simulink model "Electrical_System_2018b_obfs"  (R2019b)
settings: Solver=VariableStepAuto  StartTime=0.0  StopTime=5  RelTol=1e-3  AbsTol=1e-3  EnableMultiTasking=on
InitFcn:
  | Steady_State_Initialisation;
StopFcn:
  | %sscexplore(simlog);
  | %Logging
undefined symbols (not defined in the file): abrlhklxvp, aexgmhuedq, afmfmjnutg, afpphrjpnc, ahuxbyvruc, alarvljztt, amxnyqmnuw, aodrlwvqie, aolhmuplyq, aqpmguuqkg, auesgwirzl, aurophlnng, awamelrhru, ayfhvxflxn, azxkacuhqc, babszerikg, bawhdqanwq, bevoqecvei, bltjvqbchx, bmqsuewujl, bsmyqjfgnf, btvjbsmnve, bywgxqeadw, bziaduxaer, bzmcmdqocb, bzsvyvetat, ccsjnrbsih, cdvenygxwh, cedkrnslhx, cjheorclzs, cjrdshrtqx, ckhavyhcza, ckxewznhlz, cmrcgyiplk, conenicnws, cqkejbgjnn, csfnuwymhe, cunupkhwbh, cwzfvzuxxh, dcadmadufn, dcfponivnv, ddtrqjrhjn, dfhoxvkqas, dfrhtcwpne, dfvomcagjv, djijwylxea, dnmeqksrrm, dnzewbdkaa, dsqcykyxav, dtswwlttmm, ecumpidjtv, edegaywrct, ejjjsmnejc, eknqnehjdz, emvdetzouf, esxbqkbahr, etnkkbreiq, eunoiiiirw, ewewcuedir, fatkfxdhtc ... (+386)
libraries: fl_lib x802, ee_lib x362, fl_ps_legacy_lib x160, nesl_utility x85
(part 22 of 26)

== system Electrical_System_2018b_obfs/Redacted_1221/Redacted_7996/Redacted_9242/Redacted_38/Redacted_8107/Redacted_1499 ==
  Redacted_1372 : ee_lib/Semiconductors & Converters/Diode  ModelType=oeqafphldn  Vf=acjyupqtkx V  Ron=elvzancpcm Ohm  Goff=tujcoycxin S  prmExp=bgjswghdna  I12=bkqlogkrkf A  V12=txryfvebun V  IS=otlkguyesn A  ec=opcxekgwui  I1=zxnbsfujxu A  V1=yojkkxomec V  RS=wnxklyqkqh Ohm  Tmeas=naqktatbix degC  N_series=uibfkpxvyo  N_parallel=fsxsmxmqhq  Rz=rxievfeusi Ohm  BV=qlteerppyi V  C_param=lprewekluz  CJ=zephenugoj pF  CJ0=iofcpdtcpe pF  VJ=weostsqpeg V  Mgrad=dsfoutwajc  Vvec=nvjoneietm V  Cvec=yywdcfvqfn pF  FC=zxojfigesc  Q_param=knpwgwovvc  iRM=iptauvkfjs A  iF=evcrxohzeb A  didt=mfkykpnqxj A/us  trr_factor=dkzjtrbhin  trr=egudynmhcl ns  Qrr=skptoxjvyi s*uA  TT=uuwdjlqntv ns  tau=eybdzjqrqe ns  T_param=pdzhxnzkkw  IS_T2=skzmvmtovf A  I1_T2=bcuatdrmea A  V1_T2=ehajjhlbmz V  Tmeas2=tvtzgdgotp degC  EG_param=cqgdiwgdoz  EG=zrtjxhevif eV  XTI_param=fwomuyxozs  XTI=gvlipjngtx  dBVdT=ivbqiupcvu V/K  Tdevice=masylhgtas degC  i_specify=off  i_priority=None  i=lkqqibkans A  i_nominal_specify=off  i_nominal_unit=A  i_nominal_value=rbdmnlhukn  v_specify=off  v_priority=None  v=qqtssrhlfx V  v_nominal_specify=off  v_nominal_unit=V  v_nominal_value=qvmmnhekqw  i_capacitor_specify=off  i_capacitor_priority=None  i_capacitor=uvyrukywri A  i_capacitor_nominal_specify=off  i_capacitor_nominal_unit=A  i_capacitor_nominal_value=aribpcxhol  v_capacitor_specify=off  v_capacitor_priority=None  v_capacitor=qvaywhhawz V  v_capacitor_nominal_specify=off  v_capacitor_nominal_unit=V  v_capacitor_nominal_value=vctwyhqhyz  power_dissipated_specify=off  power_dissipated_priority=None  power_dissipated=ufpbyxefif W  power_dissipated_nominal_specify=off  power_dissipated_nominal_unit=W  power_dissipated_nominal_value=ncmyqqgdsj  thermal_network_parameterization=czsqgtsyze  Rth=deuanxgwux K/W  Rth_Foster=uzfbyrcyqk K/W  thermal_mass_parameterization=cxaszulvyr  thermal_mass=vusczqtjvo J/K  thermal_mass_Foster=bhxnhdayyv J/K  thermal_time_constant=qwdbemvqjo s  thermal_time_constant_Foster=awjktewxjv s  thermal_mass_initial_temperatures=twqhspyowt degC
      settings: SourceProductName=Simscape Electrical  InternalSimscapePortConfiguration="{\"Bottom\":[],\"Left\":[{\"id\":\"p\",\"label\":\"\",\"type\":\"foundation.electrical.electrical\"},{\"id\":\"H\",\"label\":\"H\",\"type\":\"foundation.thermal.thermal\"}],\"Right\":[{\"id\":\"n\",\"label\":\"\",\"type\":\"foundation.electrical.electrical\"}],\"Top\":[]}"
  Redacted_1419 : ee_lib/Passive/Thermal/Thermal Resistor  R=hrqrqmvbpy K/W  T_specify=off  T_priority=None  T=uzgwdnympr K  T_nominal_specify=off  T_nominal_unit=K  T_nominal_value=odnnmyuyup  Q_specify=off  Q_priority=None  Q=wmfrhtzhrt W  Q_nominal_specify=off  Q_nominal_unit=W  Q_nominal_value=ndjluapxpa
      settings: SourceProductName=Simscape Electrical  SourceProductBaseCode=PS  InternalSimscapePortConfiguration="{\"Bottom\":[],\"Left\":[{\"id\":\"A\",\"label\":\"A\",\"type\":\"foundation.thermal.thermal\"}],\"Right\":[{\"id\":\"B\",\"label\":\"B\",\"type\":\"foundation.thermal.thermal\"}],\"Top\":[]}"
  Redacted_1590 : fl_lib/Electrical/Electrical Elements/Switch  R_closed=iowuptsgqe Ohm  G_open=rxiunnesbo 1/Ohm  Threshold=unqgawnmpv  i_specify=off  i_priority=None  i=lnylkdbegy A  i_nominal_specify=off  i_nominal_unit=A  i_nominal_value=bydoewdomm  v_specify=off  v_priority=None  v=zmzvkflwcv V  v_nominal_specify=off  v_nominal_unit=V  v_nominal_value=wpiupjsgpl
      settings: SourceProductName=Simscape
  Redacted_2472 : fl_lib/Electrical/Electrical Elements/Switch  R_closed=audksowpzp Ohm  G_open=pwftaacglf 1/Ohm  Threshold=wrinmgjiem  i_specify=off  i_priority=None  i=yfbhuvnast A  i_nominal_specify=off  i_nominal_unit=A  i_nominal_value=umzifsynlf  v_specify=off  v_priority=None  v=pbbfyzmewz V  v_nominal_specify=off  v_nominal_unit=V  v_nominal_value=plmrfjgleq
      settings: SourceProductName=Simscape
  Redacted_2589 : ee_lib/Semiconductors & Converters/Diode  ModelType=rjpnrtdgtt  Vf=xzmjkgpdey V  Ron=nxlwttfate Ohm  Goff=lnyhvfbbtu S  prmExp=vonpdctgdj  I12=grmvoudklk A  V12=hqonboqbit V  IS=kmplhtdszg A  ec=tcvvdwughg  I1=fgrepgwzdh A  V1=cotflruesc V  RS=zahvsomfvl Ohm  Tmeas=vmjjndtctt degC  N_series=xsnjmnbvwt  N_parallel=nnlxfgcroq  Rz=tlllfmdkwy Ohm  BV=httyhdpdvn V  C_param=wdzgujpwis  CJ=navvsqyviu pF  CJ0=lshwbmfmpz pF  VJ=yneykywyqj V  Mgrad=iyckipozhp  Vvec=qdlpdffjte V  Cvec=qrapuwalex pF  FC=bigsaqskak  Q_param=uxgogovwjr  iRM=syhvjfhybk A  iF=kxtzgmdxyw A  didt=jnjthztocr A/us  trr_factor=tjmggzxpke  trr=vhsdneaydn ns  Qrr=tnjmgwczvn s*uA  TT=fwgrbgxdwi ns  tau=ihydaexyqv ns  T_param=lvganenigi  IS_T2=gbnfpovmzw A  I1_T2=pabzxbmlcc A  V1_T2=wqxdpehoje V  Tmeas2=rtmqbebpzh degC  EG_param=edwzkfqmdl  EG=qyccsvvwnn eV  XTI_param=omzrrxypod  XTI=ptogfqkwam  dBVdT=davhgbfmti V/K  Tdevice=hyayizqeia degC  i_specify=off  i_priority=None  i=koltymucxn A  i_nominal_specify=off  i_nominal_unit=A  i_nominal_value=mrrsdndtie  v_specify=off  v_priority=None  v=uuzqfojbot V  v_nominal_specify=off  v_nominal_unit=V  v_nominal_value=ybwzcetsjx  i_capacitor_specify=off  i_capacitor_priority=None  i_capacitor=fyvfeuymxr A  i_capacitor_nominal_specify=off  i_capacitor_nominal_unit=A  i_capacitor_nominal_value=diyyfnbabf  v_capacitor_specify=off  v_capacitor_priority=None  v_capacitor=kqzktcbdpq V  v_capacitor_nominal_specify=off  v_capacitor_nominal_unit=V  v_capacitor_nominal_value=ksvksobaqx  power_dissipated_specify=off  power_dissipated_priority=None  power_dissipated=xkfjfeadoq W  power_dissipated_nominal_specify=off  power_dissipated_nominal_unit=W  power_dissipated_nominal_value=tiyguwtfkh  thermal_network_parameterization=vzwgifhjhn  Rth=fsluxrlfjd K/W  Rth_Foster=rjdsgdjmek K/W  thermal_mass_parameterization=fpfqazpetd  thermal_mass=ajflxmskts J/K  thermal_mass_Foster=sxzzzhxfga J/K  thermal_time_constant=ajtxpvtrnh s  thermal_time_constant_Foster=wlzccrevze s  thermal_mass_initial_temperatures=yrvkmkfslp degC
      settings: SourceProductName=Simscape Electrical  InternalSimscapePortConfiguration="{\"Bottom\":[],\"Left\":[{\"id\":\"p\",\"label\":\"\",\"type\":\"foundation.electrical.electrical\"},{\"id\":\"H\",\"label\":\"H\",\"type\":\"foundation.thermal.thermal\"}],\"Right\":[{\"id\":\"n\",\"label\":\"\",\"type\":\"foundation.electrical.electrical\"}],\"Top\":[]}"
  Redacted_3285 : ee_lib/Passive/Thermal/Thermal Resistor  R=aexgmhuedq K/W  T_specify=off  T_priority=None  T=mjrhfjyuzy K  T_nominal_specify=off  T_nominal_unit=K  T_nominal_value=vddbbbtjss  Q_specify=off  Q_priority=None  Q=sstmdjjadm W  Q_nominal_specify=off  Q_nominal_unit=W  Q_nominal_value=fgusrenltz
      settings: SourceProductName=Simscape Electrical  SourceProductBaseCode=PS  InternalSimscapePortConfiguration="{\"Bottom\":[],\"Left\":[{\"id\":\"A\",\"label\":\"A\",\"type\":\"foundation.thermal.thermal\"}],\"Right\":[{\"id\":\"B\",\"label\":\"B\",\"type\":\"foundation.thermal.thermal\"}],\"Top\":[]}"
  Redacted_3696 : ee_lib/Passive/Thermal/Thermal Resistor  R=glalizypuy K/W  T_specify=off  T_priority=None  T=muvcehmgvy K  T_nominal_specify=off  T_nominal_unit=K  T_nominal_value=iimdorgzkx  Q_specify=off  Q_priority=None  Q=ksqhixmxvw W  Q_nominal_specify=off  Q_nominal_unit=W  Q_nominal_value=szsgvwogcu
      settings: SourceProductName=Simscape Electrical  SourceProductBaseCode=PS  InternalSimscapePortConfiguration="{\"Bottom\":[],\"Left\":[{\"id\":\"A\",\"label\":\"A\",\"type\":\"foundation.thermal.thermal\"}],\"Right\":[{\"id\":\"B\",\"label\":\"B\",\"type\":\"foundation.thermal.thermal\"}],\"Top\":[]}"
  Redacted_4558 : fl_lib/Electrical/Electrical Elements/Switch  R_closed=asjgucvpwv Ohm  G_open=frheikthvf 1/Ohm  Threshold=gvgivrruxe  i_specify=off  i_priority=None  i=awnvafosau A  i_nominal_specify=off  i_nominal_unit=A  i_nominal_value=kbahxsqmia  v_specify=off  v_priority=None  v=fmojvofggq V  v_nominal_specify=off  v_nominal_unit=V  v_nominal_value=hpesrfkdpt
      settings: SourceProductName=Simscape
  Redacted_642 : ee_lib/Semiconductors & Converters/Diode  ModelType=zgqjdnfvyg  Vf=krhvtwcfjx V  Ron=ltlocceomt Ohm  Goff=hvgqhqmuzj S  prmExp=knqxglupvh  I12=wjgwkrterc A  V12=iehppplrze V  IS=cllsdmmlqs A  ec=iucoqlglyn  I1=shzivgnrjs A  V1=vvxsvbngjn V  RS=hxvfllnfuh Ohm  Tmeas=dreqftvwty degC  N_series=bgchqtupvy  N_parallel=kffrtauvvf  Rz=leoaehqcru Ohm  BV=jcblpiykgg V  C_param=nueawtycbx  CJ=yafxcafril pF  CJ0=hbcrilffht pF  VJ=mwtcezhpyo V  Mgrad=xptgjoikwd  Vvec=zrohyynisq V  Cvec=ppfbuygtgp pF  FC=vtobxydlyp  Q_param=qkiyqbzmmd  iRM=vvnzrrctjv A  iF=ahyfmbtmnp A  didt=hikchliuiw A/us  trr_factor=qmqajofqif  trr=rqfqsucxvw ns  Qrr=jzeozeaxkq s*uA  TT=owzzigtdqq ns  tau=dkiwhaezua ns  T_param=drpeomdfld  IS_T2=uvjoyzqlmj A  I1_T2=jjcpkvqtxo A  V1_T2=pahhbigbow V  Tmeas2=qljyojmmfe degC  EG_param=nxiorexete  EG=addbzoglki eV  XTI_param=bwvlanfros  XTI=orqisdqqcy  dBVdT=qecfhbpvnf V/K  Tdevice=umhofmsqaj degC  i_specify=off  i_priority=None  i=uhnhxgwkyy A  i_nominal_specify=off  i_nominal_unit=A  i_nominal_value=rwbjerovzq  v_specify=off  v_priority=None  v=unbgguzoer V  v_nominal_specify=off  v_nominal_unit=V  v_nominal_value=bsojsposnt  i_capacitor_specify=off  i_capacitor_priority=None  i_capacitor=jwkadmeyvr A  i_capacitor_nominal_specify=off  i_capacitor_nominal_unit=A  i_capacitor_nominal_value=aljrhofyuz  v_capacitor_specify=off  v_capacitor_priority=None  v_capacitor=piziulizqv V  v_capacitor_nominal_specify=off  v_capacitor_nominal_unit=V  v_capacitor_nominal_value=oygxflyfjn  power_dissipated_specify=off  power_dissipated_priority=None  power_dissipated=cggjjryskq W  power_dissipated_nominal_specify=off  power_dissipated_nominal_unit=W  power_dissipated_nominal_value=kljlgaczdh  thermal_network_parameterization=hzdelgpiuu  Rth=cugitvfnne K/W  Rth_Foster=wfsuulygfd K/W  thermal_mass_parameterization=umberrvwxd  thermal_mass=mssuiqenen J/K  thermal_mass_Foster=ydktevffor J/K  thermal_time_constant=vvxxixcgsx s  thermal_time_constant_Foster=gljfbbzout s  thermal_mass_initial_temperatures=niolpbupdj degC
      settings: SourceProductName=Simscape Electrical  InternalSimscapePortConfiguration="{\"Bottom\":[],\"Left\":[{\"id\":\"p\",\"label\":\"\",\"type\":\"foundation.electrical.electrical\"},{\"id\":\"H\",\"label\":\"H\",\"type\":\"foundation.thermal.thermal\"}],\"Right\":[{\"id\":\"n\",\"label\":\"\",\"type\":\"foundation.electrical.electrical\"}],\"Top\":[]}"
  Redacted_6679 : ee_lib/Semiconductors & Converters/Diode  ModelType=hfoamrqohn  Vf=ymdzzcsmqr V  Ron=atfpidzbvs Ohm  Goff=wlfmjvgosd S  prmExp=tkyrtviuba  I12=ijhixfgdxe A  V12=pzriwjhaus V  IS=smuzhnhjiq A  ec=anazatfevq  I1=wfziekknxg A  V1=rqdikadhpp V  RS=fmeqsuvzaj Ohm  Tmeas=wquurlonrk degC  N_series=xvlhvgawtc  N_parallel=fybtoxfnlt  Rz=zzlhcdkaxf Ohm  BV=kctcbwnpgv V  C_param=sbntavnrmi  CJ=eksdzpdgwu pF  CJ0=dhieudjrsd pF  VJ=tvpzscfnfd V  Mgrad=odrhjhrowr  Vvec=lvmxtkcqsx V  Cvec=aooufnefqf pF  FC=xgngsjjuyq  Q_param=tdleidmezo  iRM=shidknspef A  iF=wywaxscsxu A  didt=uoogvgzytp A/us  trr_factor=mvjcgsflfu  trr=hcmpjhwool ns  Qrr=hlpbbzpaoi s*uA  TT=nenlhgdgft ns  tau=vpgivdtofh ns  T_param=bxtgxeurxd  IS_T2=dsopsgnyjc A  I1_T2=wnefpaqyvx A  V1_T2=tgewoyoysb V  Tmeas2=dowbkkuwwl degC  EG_param=wiplfunvyd  EG=ehkmoclttv eV  XTI_param=spldrpwhzd  XTI=bsukslgsxi  dBVdT=wlzooyfsxr V/K  Tdevice=vnwykbyqrk degC  i_specify=off  i_priority=None  i=ldwgybfoxv A  i_nominal_specify=off  i_nominal_unit=A  i_nominal_value=zenvsgodqo  v_specify=off  v_priority=None  v=wnlnxjdwgs V  v_nominal_specify=off  v_nominal_unit=V  v_nominal_value=rpaaihxlse  i_capacitor_specify=off  i_capacitor_priority=None  i_capacitor=imcsdhdxqi A  i_capacitor_nominal_specify=off  i_capacitor_nominal_unit=A  i_capacitor_nominal_value=cwpbaclfsw  v_capacitor_specify=off  v_capacitor_priority=None  v_capacitor=dmlqioyezl V  v_capacitor_nominal_specify=off  v_capacitor_nominal_unit=V  v_capacitor_nominal_value=ivivdmncvx  power_dissipated_specify=off  power_dissipated_priority=None  power_dissipated=ffhvkzmmzr W  power_dissipated_nominal_specify=off  power_dissipated_nominal_unit=W  power_dissipated_nominal_value=jhrvkhwpck  thermal_network_parameterization=chcnnnqdvq  Rth=typqmdcyob K/W  Rth_Foster=cclidkkojd K/W  thermal_mass_parameterization=fufscafdar  thermal_mass=rrtwbudeji J/K  thermal_mass_Foster=flntkiygyu J/K  thermal_time_constant=ewfqvootyi s  thermal_time_constant_Foster=uzgtcdfumv s  thermal_mass_initial_temperatures=xiusirosom degC
      settings: SourceProductName=Simscape Electrical  InternalSimscapePortConfiguration="{\"Bottom\":[],\"Left\":[{\"id\":\"p\",\"label\":\"\",\"type\":\"foundation.electrical.electrical\"},{\"id\":\"H\",\"label\":\"H\",\"type\":\"foundation.thermal.thermal\"}],\"Right\":[{\"id\":\"n\",\"label\":\"\",\"type\":\"foundation.electrical.electrical\"}],\"Top\":[]}"
  Redacted_6984 : ee_lib/Semiconductors & Converters/Diode  ModelType=dbxjdtelfg  Vf=jrlektwyix V  Ron=vkbbnnynsg Ohm  Goff=yuuxvmfwgf S  prmExp=fyuvcmxyra  I12=tlbhcqdpkd A  V12=tklehtcaqc V  IS=slukjhdrqy A  ec=atwalcumyw  I1=vxrhtljmne A  V1=bjeljqtgdd V  RS=odobhiftnb Ohm  Tmeas=uhoqtneexa degC  N_series=etmbfinxuu  N_parallel=rqyiffyciq  Rz=msphxnvwlx Ohm  BV=lrusecstot V  C_param=ngtamvhrla  CJ=hqvnfakstq pF  CJ0=wvvnorcllh pF  VJ=mbkuzfaafy V  Mgrad=rrumwpgudm  Vvec=lwljdgvidx V  Cvec=qvcxokabqx pF  FC=lppqiohzlu  Q_param=ocbqtiivdt  iRM=ietiqfrqdc A  iF=flngrbuzfp A  didt=frfvuotyji A/us  trr_factor=qbakmbcuuz  trr=rkkgbwgnpq ns  Qrr=prcotekwhx s*uA  TT=fbcfdtvgnr ns  tau=ivfqbbawng ns  T_param=yvmphdqqpd  IS_T2=jaijzlblcu A  I1_T2=hpvlwpoizb A  V1_T2=rlynjzjkuy V  Tmeas2=tptbqblhfe degC  EG_param=yzlvjciftk  EG=nxgiyokdrm eV  XTI_param=krckmpusmp  XTI=cnjttxxpvy  dBVdT=nxuivboalv V/K  Tdevice=vjhlnzzfra degC  i_specify=off  i_priority=None  i=xvetthaiff A  i_nominal_specify=off  i_nominal_unit=A  i_nominal_value=bxbqqumvtn  v_specify=off  v_priority=None  v=avotebfbkl V  v_nominal_specify=off  v_nominal_unit=V  v_nominal_value=vmpuezgydd  i_capacitor_specify=off  i_capacitor_priority=None  i_capacitor=ijlvjdjbhu A  i_capacitor_nominal_specify=off  i_capacitor_nominal_unit=A  i_capacitor_nominal_value=vrexwqbbfc  v_capacitor_specify=off  v_capacitor_priority=None  v_capacitor=bzetwmwljd V  v_capacitor_nominal_specify=off  v_capacitor_nominal_unit=V  v_capacitor_nominal_value=oqhagsuuvs  power_dissipated_specify=off  power_dissipated_priority=None  power_dissipated=zkwrxanbch W  power_dissipated_nominal_specify=off  power_dissipated_nominal_unit=W  power_dissipated_nominal_value=ptbptrhtfc  thermal_network_parameterization=irgsgxwqnd  Rth=usshznhwqn K/W  Rth_Foster=reibnptawl K/W  thermal_mass_parameterization=xcjefrmilo  thermal_mass=yjcjigqudt J/K  thermal_mass_Foster=jmrnevjoro J/K  thermal_time_constant=acvfifvwfh s  thermal_time_constant_Foster=gpfpiqslez s  thermal_mass_initial_temperatures=qvznhxjxbn degC
      settings: SourceProductName=Simscape Electrical  InternalSimscapePortConfiguration="{\"Bottom\":[],\"Left\":[{\"id\":\"p\",\"label\":\"\",\"type\":\"foundation.electrical.electrical\"},{\"id\":\"H\",\"label\":\"H\",\"type\":\"foundation.thermal.thermal\"}],\"Right\":[{\"id\":\"n\",\"label\":\"\",\"type\":\"foundation.electrical.electrical\"}],\"Top\":[]}"
  Redacted_8398 : ee_lib/Passive/Thermal/Thermal Resistor  R=mjpoozxhec K/W  T_specify=off  T_priority=None  T=babszerikg K  T_nominal_specify=off  T_nominal_unit=K  T_nominal_value=nwfssbnthp  Q_specify=off  Q_priority=None  Q=nkxxqhugfh W  Q_nominal_specify=off  Q_nominal_unit=W  Q_nominal_value=waicngwfjd
      settings: SourceProductName=Simscape Electrical  SourceProductBaseCode=PS  InternalSimscapePortConfiguration="{\"Bottom\":[],\"Left\":[{\"id\":\"A\",\"label\":\"A\",\"type\":\"foundation.thermal.thermal\"}],\"Right\":[{\"id\":\"B\",\"label\":\"B\",\"type\":\"foundation.thermal.thermal\"}],\"Top\":[]}"
  Redacted_3847 : PMIOPort  Side=Left
  Redacted_7258 : PMIOPort  Port=2  Side=Left
  Redacted_9653 : PMIOPort  Port=3  Side=Left
  Redacted_8670 : PMIOPort  Port=4  Side=Right
  Redacted_1560 : PMIOPort  Port=5  Side=Right
  Redacted_5472 : PMIOPort  Port=6  Side=Right
  Redacted_6523 : PMIOPort  Port=7  Side=Left
  Redacted_5320 : PMIOPort  Port=8  Side=Right
  connections:
  Redacted_2589/LConn2 -- Redacted_3696/LConn1
  Redacted_3285/RConn1 -- Redacted_6523/RConn1
  Redacted_6984/LConn2 -- Redacted_1419/LConn1 -- Redacted_1372/LConn2
  Redacted_6984/RConn1 -- Redacted_1590/LConn1 -- Redacted_1372/LConn1
  Redacted_1560/RConn1 -- Redacted_2472/RConn2
  Redacted_4558/RConn1 -- Redacted_2472/RConn1 -- Redacted_1590/RConn1 -- Redacted_5320/RConn1
  Redacted_5472/RConn1 -- Redacted_1590/RConn2
  Redacted_1372/RConn1 -- Redacted_9653/RConn1 -- Redacted_6984/LConn1
  Redacted_3285/LConn1 -- Redacted_1419/RConn1 -- Redacted_8398/RConn1 -- Redacted_3696/RConn1
  Redacted_642/RConn1 -- Redacted_3847/RConn1 -- Redacted_6679/LConn1
  Redacted_6679/RConn1 -- Redacted_4558/LConn1 -- Redacted_642/LConn1
  Redacted_8670/RConn1 -- Redacted_4558/RConn2
  Redacted_642/LConn2 -- Redacted_6679/LConn2 -- Redacted_8398/LConn1
  Redacted_2589/RConn1 -- Redacted_2472/LConn1
  Redacted_2589/LConn1 -- Redacted_7258/RConn1

== system Electrical_System_2018b_obfs/Redacted_1221/Redacted_7996/Redacted_9242/Redacted_38/Redacted_8107/Redacted_3070 ==
  Neutral_Negative : Subsystem  VariantControl=Variant1
  Positive_Neutral : Subsystem  VariantControl=Variant3
  Redacted_6581 : Subsystem  VariantControl=Variant2
  Redacted_9800 : PMIOPort  Side=Left
  Redacted_6600 : PMIOPort  Port=2  Side=Left
  Redacted_5239 : PMIOPort  Port=3  Side=Left
  Redacted_3081 : PMIOPort  Port=4  Side=Right
  Redacted_7642 : PMIOPort  Port=5  Side=Right

== system Electrical_System_2018b_obfs/Redacted_1221/Redacted_7996/Redacted_9242/Redacted_38/Redacted_8107/Redacted_4713 ==
  Redacted_1933 : ee_lib/Passive/Thermal/Thermal Resistor  R=vqzdbndqcq K/W  T_specify=off  T_priority=None  T=nqnzssezxm K  T_nominal_specify=off  T_nominal_unit=K  T_nominal_value=lsoyswnfcd  Q_specify=off  Q_priority=None  Q=gcpbocbgtt W  Q_nominal_specify=off  Q_nominal_unit=W  Q_nominal_value=vtffvadatd
      settings: SourceProductName=Simscape Electrical  SourceProductBaseCode=PS  InternalSimscapePortConfiguration="{\"Bottom\":[],\"Left\":[{\"id\":\"A\",\"label\":\"A\",\"type\":\"foundation.thermal.thermal\"}],\"Right\":[{\"id\":\"B\",\"label\":\"B\",\"type\":\"foundation.thermal.thermal\"}],\"Top\":[]}"
  Redacted_5420 : ee_lib/Passive/Thermal/Thermal Resistor  R=xmufvapubo K/W  T_specify=off  T_priority=None  T=ecumpidjtv K  T_nominal_specify=off  T_nominal_unit=K  T_nominal_value=lvwljextpv  Q_specify=off  Q_priority=None  Q=vwqjenfcut W  Q_nominal_specify=off  Q_nominal_unit=W  Q_nominal_value=cixwplaltu
      settings: SourceProductName=Simscape Electrical  SourceProductBaseCode=PS  InternalSimscapePortConfiguration="{\"Bottom\":[],\"Left\":[{\"id\":\"A\",\"label\":\"A\",\"type\":\"foundation.thermal.thermal\"}],\"Right\":[{\"id\":\"B\",\"label\":\"B\",\"type\":\"foundation.thermal.thermal\"}],\"Top\":[]}"
  Redacted_5860 : ee_lib/Semiconductors & Converters/Diode  ModelType=wsmsvgvpjr  Vf=ggtrbonwka V  Ron=klzenpjchx Ohm  Goff=afeiecyrvl S  prmExp=wjpvzuidnm  I12=nzrdqjbudh A  V12=juwlmthuyi V  IS=hoasnoacdd A  ec=iglqywrysv  I1=fhrwoxdfcq A  V1=fyrsqtuyea V  RS=cwkauqcaqf Ohm  Tmeas=wslazedzuw degC  N_series=xayqvkljdg  N_parallel=mcglifjfpj  Rz=cdpoolaiug Ohm  BV=mwrqkpwyun V  C_param=yyprdzpkjg  CJ=wpcjqojxlz pF  CJ0=qmeglslxxj pF  VJ=djcigfteis V  Mgrad=ougvijtmes  Vvec=lqbbwnorbm V  Cvec=nlilfjfqpv pF  FC=klnwovienj  Q_param=kxlwvyopnt  iRM=sddcsiesyi A  iF=pijofqeilq A  didt=hnawmoexou A/us  trr_factor=tivakyulur  trr=awpjflknij ns  Qrr=wnewuritje s*uA  TT=vqopymrgup ns  tau=bkqagddhtq ns  T_param=ltcpgxqdhc  IS_T2=dstotmvkwn A  I1_T2=iymegpyqie A  V1_T2=umpoeincal V  Tmeas2=kmpwxudgqu degC  EG_param=sruxebchkg  EG=nkijjvyhdb eV  XTI_param=ufjalowwbi  XTI=zuhdzluwar  dBVdT=wtvroynkhd V/K  Tdevice=etzodnxspp degC  i_specify=off  i_priority=None  i=ucztdhflhm A  i_nominal_specify=off  i_nominal_unit=A  i_nominal_value=xkjtclnfqg  v_specify=off  v_priority=None  v=nbqnomyygd V  v_nominal_specify=off  v_nominal_unit=V  v_nominal_value=fzzxmdvcok  i_capacitor_specify=off  i_capacitor_priority=None  i_capacitor=jqgxtsrgle A  i_capacitor_nominal_specify=off  i_capacitor_nominal_unit=A  i_capacitor_nominal_value=vkazerubet  v_capacitor_specify=off  v_capacitor_priority=None  v_capacitor=ebcphkcsez V  v_capacitor_nominal_specify=off  v_capacitor_nominal_unit=V  v_capacitor_nominal_value=prfjatkoki  power_dissipated_specify=off  power_dissipated_priority=None  power_dissipated=pguckrmjzv W  power_dissipated_nominal_specify=off  power_dissipated_nominal_unit=W  power_dissipated_nominal_value=qbzdzdtwwv  thermal_network_parameterization=xmrqnfmybs  Rth=elkydoragp K/W  Rth_Foster=obqeloajzd K/W  thermal_mass_parameterization=xcultdbsju  thermal_mass=oevkquafmk J/K  thermal_mass_Foster=kdignddeuh J/K  thermal_time_constant=lwnmdhsgez s  thermal_time_constant_Foster=erfxczdcji s  thermal_mass_initial_temperatures=yttjglblsu degC
      settings: SourceProductName=Simscape Electrical  InternalSimscapePortConfiguration="{\"Bottom\":[],\"Left\":[{\"id\":\"p\",\"label\":\"\",\"type\":\"foundation.electrical.electrical\"},{\"id\":\"H\",\"label\":\"H\",\"type\":\"foundation.thermal.thermal\"}],\"Right\":[{\"id\":\"n\",\"label\":\"\",\"type\":\"foundation.electrical.electrical\"}],\"Top\":[]}"
  Redacted_5973 : ee_lib/Semiconductors & Converters/Diode  ModelType=grmprtzwjb  Vf=yhddqqrndc V  Ron=jlwcbxzdvc Ohm  Goff=uencbjsfad S  prmExp=oodxnndica  I12=ebnuqqlinq A  V12=jfwqutoswe V  IS=emditcitqg A  ec=frnzgashys  I1=txytnqqupz A  V1=ctwajydwez V  RS=kqbbfucwyp Ohm  Tmeas=xgbttyyimn degC  N_series=qiramoyclr  N_parallel=lsqpqduyim  Rz=vvqnlmazkn Ohm  BV=obpwncwyqf V  C_param=toribicxvy  CJ=mfwgegjbqv pF  CJ0=sexloyujjy pF  VJ=giykssekkn V  Mgrad=ayqdpgyqam  Vvec=alunubzrbl V  Cvec=odwvkdcuef pF  FC=aeaflmriwc  Q_param=fhilakndnd  iRM=iraaaecfcn A  iF=xitbpyfhkw A  didt=gqauvmekcu A/us  trr_factor=rtdqckoflm  trr=dajbhvonqc ns  Qrr=tlxzgpawqu s*uA  TT=gmgvpxnoge ns  tau=zwrshxbeio ns  T_param=csbtzfytly  IS_T2=nwohxaibmu A  I1_T2=fzkcnxadkh A  V1_T2=uiphwpxdwt V  Tmeas2=ltwwpwbepu degC  EG_param=uqvtfzgaei  EG=snkjuqejab eV  XTI_param=ogqsjulyvm  XTI=cseqsougqi  dBVdT=leeitqmrpj V/K  Tdevice=yrdonghwpo degC  i_specify=off  i_priority=None  i=yhnbftkohk A  i_nominal_specify=off  i_nominal_unit=A  i_nominal_value=cjalikrmpp  v_specify=off  v_priority=None  v=skiwotjvvl V  v_nominal_specify=off  v_nominal_unit=V  v_nominal_value=ujhxnbkruz  i_capacitor_specify=off  i_capacitor_priority=None  i_capacitor=idfehlvdwr A  i_capacitor_nominal_specify=off  i_capacitor_nominal_unit=A  i_capacitor_nominal_value=sctzqilkri  v_capacitor_specify=off  v_capacitor_priority=None  v_capacitor=htyzmhhlrg V  v_capacitor_nominal_specify=off  v_capacitor_nominal_unit=V  v_capacitor_nominal_value=cvcknlawah  power_dissipated_specify=off  power_dissipated_priority=None  power_dissipated=wuexpqnevc W  power_dissipated_nominal_specify=off  power_dissipated_nominal_unit=W  power_dissipated_nominal_value=vqotlhnjum  thermal_network_parameterization=zpcslduydh  Rth=jfyaocrmdt K/W  Rth_Foster=eugapkemnj K/W  thermal_mass_parameterization=yxhowqnhjx  thermal_mass=hjpmphgocn J/K  thermal_mass_Foster=dehjnwgqho J/K  thermal_time_constant=txykdimmdy s  thermal_time_constant_Foster=hbxohydkpe s  thermal_mass_initial_temperatures=ctyzphvplu degC
      settings: SourceProductName=Simscape Electrical  InternalSimscapePortConfiguration="{\"Bottom\":[],\"Left\":[{\"id\":\"p\",\"label\":\"\",\"type\":\"foundation.electrical.electrical\"},{\"id\":\"H\",\"label\":\"H\",\"type\":\"foundation.thermal.thermal\"}],\"Right\":[{\"id\":\"n\",\"label\":\"\",\"type\":\"foundation.electrical.electrical\"}],\"Top\":[]}"
  Redacted_6743 : fl_lib/Electrical/Electrical Elements/Switch  R_closed=uirsufpzgz Ohm  G_open=mhxpckfjeh 1/Ohm  Threshold=lllvbipbnz  i_specify=off  i_priority=None  i=rrctbvjnhf A  i_nominal_specify=off  i_nominal_unit=A  i_nominal_value=erijjpysit  v_specify=off  v_priority=None  v=bmormrfokg V  v_nominal_specify=off  v_nominal_unit=V  v_nominal_value=eroebjzxcx
      settings: SourceProductName=Simscape
  Redacted_7227 : ee_lib/Passive/Thermal/Thermal Resistor  R=vrvhqtuogs K/W  T_specify=off  T_priority=None  T=tvgwlekxkg K  T_nominal_specify=off  T_nominal_unit=K  T_nominal_value=obtvfwsmke  Q_specify=off  Q_priority=None  Q=tbcalngzwi W  Q_nominal_specify=off  Q_nominal_unit=W  Q_nominal_value=zgszgiaxcq
      settings: SourceProductName=Simscape Electrical  SourceProductBaseCode=PS  InternalSimscapePortConfiguration="{\"Bottom\":[],\"Left\":[{\"id\":\"A\",\"label\":\"A\",\"type\":\"foundation.thermal.thermal\"}],\"Right\":[{\"id\":\"B\",\"label\":\"B\",\"type\":\"foundation.thermal.thermal\"}],\"Top\":[]}"
  Redacted_7604 : ee_lib/Passive/Thermal/Thermal Resistor  R=tdkykuglzg K/W  T_specify=off  T_priority=None  T=gcfqhvdsfj K  T_nominal_specify=off  T_nominal_unit=K  T_nominal_value=fdmurrxshp  Q_specify=off  Q_priority=None  Q=kaqdrwkoog W  Q_nominal_specify=off  Q_nominal_unit=W  Q_nominal_value=mipfaifrtb
      settings: SourceProductName=Simscape Electrical  SourceProductBaseCode=PS  InternalSimscapePortConfiguration="{\"Bottom\":[],\"Left\":[{\"id\":\"A\",\"label\":\"A\",\"type\":\"foundation.thermal.thermal\"}],\"Right\":[{\"id\":\"B\",\"label\":\"B\",\"type\":\"foundation.thermal.thermal\"}],\"Top\":[]}"
  Redacted_7644 : fl_lib/Electrical/Electrical Elements/Switch  R_closed=pvhuxnurni Ohm  G_open=gtjgjewndg 1/Ohm  Threshold=aurophlnng  i_specify=off  i_priority=None  i=ofrntyceth A  i_nominal_specify=off  i_nominal_unit=A  i_nominal_value=ngawfluacd  v_specify=off  v_priority=None  v=atkfeqnsxe V  v_nominal_specify=off  v_nominal_unit=V  v_nominal_value=rgxrcyakqf
      settings: SourceProductName=Simscape
  Redacted_7937 : ee_lib/Semiconductors & Converters/Diode  ModelType=oyshwfuekh  Vf=gihuyznhrq V  Ron=hdtmjbvekb Ohm  Goff=gybtmkfjbr S  prmExp=xgqxklnndv  I12=gdarpsdlgh A  V12=hphgqxlxof V  IS=jenzsmzvmp A  ec=jokopeubjy  I1=ltokkvbyoz A  V1=avqnmwzvck V  RS=lkdsrgjcvt Ohm  Tmeas=sehftnjsmm degC  N_series=jmbuymvoul  N_parallel=gunertpuef  Rz=rwuvvfevxg Ohm  BV=xdbnwkdovz V  C_param=bpwqmhgsxz  CJ=plquocbmtv pF  CJ0=skzbnhltiy pF  VJ=mdcwqnnnfo V  Mgrad=htlxuhxsld  Vvec=dsuilgegmy V  Cvec=aojhhpfkyp pF  FC=fkionwjqom  Q_param=bwyyfpidti  iRM=qozwxlltsm A  iF=publyhkdae A  didt=ufckthsifb A/us  trr_factor=wnoxcenpyj  trr=lrbvysypeu ns  Qrr=nnnzpackib s*uA  TT=dymwyuffxe ns  tau=jxosrswpyb ns  T_param=ibajmxlgwh  IS_T2=domoyratgl A  I1_T2=zznzpwveze A  V1_T2=yshjdhsflg V  Tmeas2=tmueadmbtu degC  EG_param=phbtytevmz  EG=bojpxxswqz eV  XTI_param=iihmsgrykr  XTI=lbczzgijaa  dBVdT=excjyibwli V/K  Tdevice=usedkkqpbv degC  i_specify=off  i_priority=None  i=rhcvdyklhy A  i_nominal_specify=off  i_nominal_unit=A  i_nominal_value=qgjtsfxpcw  v_specify=off  v_priority=None  v=inmoiwklul V  v_nominal_specify=off  v_nominal_unit=V  v_nominal_value=jtoosqqgtu  i_capacitor_specify=off  i_capacitor_priority=None  i_capacitor=pmqtadvnhk A  i_capacitor_nominal_specify=off  i_capacitor_nominal_unit=A  i_capacitor_nominal_value=tullxxmiht  v_capacitor_specify=off  v_capacitor_priority=None  v_capacitor=fbtqzmdsfc V  v_capacitor_nominal_specify=off  v_capacitor_nominal_unit=V  v_capacitor_nominal_value=jxkhzwnsmu  power_dissipated_specify=off  power_dissipated_priority=None  power_dissipated=rksnrnggty W  power_dissipated_nominal_specify=off  power_dissipated_nominal_unit=W  power_dissipated_nominal_value=lptdgzddmc  thermal_network_parameterization=gdjjhkseyq  Rth=cuoltxjmuz K/W  Rth_Foster=yaoatvlekf K/W  thermal_mass_parameterization=gqbuxxvfds  thermal_mass=kbblbuljfa J/K  thermal_mass_Foster=jpvkmbituc J/K  thermal_time_constant=wsfnwatwou s  thermal_time_constant_Foster=fcpuhbuemk s  thermal_mass_initial_temperatures=bkwedbwrzf degC
      settings: SourceProductName=Simscape Electrical  InternalSimscapePortConfiguration="{\"Bottom\":[],\"Left\":[{\"id\":\"p\",\"label\":\"\",\"type\":\"foundation.electrical.electrical\"},{\"id\":\"H\",\"label\":\"H\",\"type\":\"foundation.thermal.thermal\"}],\"Right\":[{\"id\":\"n\",\"label\":\"\",\"type\":\"foundation.electrical.electrical\"}],\"Top\":[]}"
  Redacted_7973 : ee_lib/Semiconductors & Converters/Diode  ModelType=bhsujtrrdp  Vf=yumzkpdaub V  Ron=jglvprmidv Ohm  Goff=uwryahxgzt S  prmExp=erarzqgnfg  I12=usfmdmbkex A  V12=mddngxmgeh V  IS=nkihwyzdsz A  ec=qjpmtqyrwm  I1=hlppzpqowj A  V1=wnkrwcyjus V  RS=jbqroqiqbn Ohm  Tmeas=aklfryvjak degC  N_series=rkobfjynvp  N_parallel=eekiwyuijv  Rz=quedlaztup Ohm  BV=czffashbla V  C_param=xboukmwvjp  CJ=nzdjlwdqob pF  CJ0=waxdbrzrtx pF  VJ=edmgkhxveo V  Mgrad=jkagadohjt  Vvec=lpjzpuwcin V  Cvec=jqqxknnoym pF  FC=exacokewog  Q_param=laqtzeouia  iRM=nngkchwgdo A  iF=euanmuvyfa A  didt=kdykghpjcg A/us  trr_factor=mbmecyeato  trr=aqhfqdgcba ns  Qrr=ghltfdlnmb s*uA  TT=ygleunduce ns  tau=dnjemzzrtd ns  T_param=ekxwpircsy  IS_T2=zdhjrespey A  I1_T2=gfkuecvccd A  V1_T2=gsyqsokssz V  Tmeas2=cooembfiqi degC  EG_param=kusxnchfqr  EG=fodgbxzrna eV  XTI_param=rblbjpzwzg  XTI=cuaqwnfobw  dBVdT=kylnxbdjmr V/K  Tdevice=rxmvaltuyf degC  i_specify=off  i_priority=None  i=juaeqpqtxx A  i_nominal_specify=off  i_nominal_unit=A  i_nominal_value=iiimngsyje  v_specify=off  v_priority=None  v=cicmbfhzrj V  v_nominal_specify=off  v_nominal_unit=V  v_nominal_value=yjwifhkxjh  i_capacitor_specify=off  i_capacitor_priority=None  i_capacitor=dfszydlupe A  i_capacitor_nominal_specify=off  i_capacitor_nominal_unit=A  i_capacitor_nominal_value=hbbgxhhrtj  v_capacitor_specify=off  v_capacitor_priority=None  v_capacitor=ntubeqzgsa V  v_capacitor_nominal_specify=off  v_capacitor_nominal_unit=V  v_capacitor_nominal_value=qatvfjupjt  power_dissipated_specify=off  power_dissipated_priority=None  power_dissipated=qybiidjcbi W  power_dissipated_nominal_specify=off  power_dissipated_nominal_unit=W  power_dissipated_nominal_value=buppnezpqh  thermal_network_parameterization=fkkirzjzxu  Rth=aqkchzuakv K/W  Rth_Foster=pckxzdasds K/W  thermal_mass_parameterization=pygceihjak  thermal_mass=wngegxbhct J/K  thermal_mass_Foster=pofsitaali J/K  thermal_time_constant=kvinpzyeem s  thermal_time_constant_Foster=uuolpykltq s  thermal_mass_initial_temperatures=jscjfxsyye degC
      settings: SourceProductName=Simscape Electrical  InternalSimscapePortConfiguration="{\"Bottom\":[],\"Left\":[{\"id\":\"p\",\"label\":\"\",\"type\":\"foundation.electrical.electrical\"},{\"id\":\"H\",\"label\":\"H\",\"type\":\"foundation.thermal.thermal\"}],\"Right\":[{\"id\":\"n\",\"label\":\"\",\"type\":\"foundation.electrical.electrical\"}],\"Top\":[]}"
  Redacted_8421 : ee_lib/Semiconductors & Converters/Diode  ModelType=jtqppajxzp  Vf=gocoasaxlm V  Ron=qcyhggoxot Ohm  Goff=dlhxgcickd S  prmExp=pxlmmfygoq  I12=wymmfmnoyx A  V12=sxhjllusdt V  IS=gmlslrmdwd A  ec=bgzhkprxyl  I1=rpysvahrye A  V1=dmmtgtemku V  RS=gsucrqqvyo Ohm  Tmeas=byuxkgehdt degC  N_series=tqgxgzsbrk  N_parallel=swxydcszbz  Rz=wfadupajon Ohm  BV=bbsgpjwuvm V  C_param=yjjqoalfpi  CJ=rgxvjxztou pF  CJ0=fxqmawlxmc pF  VJ=jrkshlsdbu V  Mgrad=ewpfwgyyxq  Vvec=hrzuxpugzr V  Cvec=smsexqjama pF  FC=vdurzwouah  Q_param=ebnzoqqwas  iRM=cuyidxodhm A  iF=tnvfxsnows A  didt=qfeiqcorjg A/us  trr_factor=tafvhwmozh  trr=nysiatgffg ns  Qrr=pjeoszzill s*uA  TT=obwcqpazqo ns  tau=xflqetxmug ns  T_param=wrbhaydtpu  IS_T2=gecrdqkmrm A  I1_T2=udzfjlqhbr A  V1_T2=iykalwfpwx V  Tmeas2=vrqwoxvpuq degC  EG_param=xnotqjssvw  EG=dixxhqlpev eV  XTI_param=fnkdvoeqxq  XTI=sobuysmbnk  dBVdT=zoaptztxwc V/K  Tdevice=pejllpfkcr degC  i_specify=off  i_priority=None  i=lurdanofgi A  i_nominal_specify=off  i_nominal_unit=A  i_nominal_value=wkkykgynbr  v_specify=off  v_priority=None  v=zjsfnwblcd V  v_nominal_specify=off  v_nominal_unit=V  v_nominal_value=jyrkwvgjuf  i_capacitor_specify=off  i_capacitor_priority=None  i_capacitor=uizsklogiq A  i_capacitor_nominal_specify=off  i_capacitor_nominal_unit=A  i_capacitor_nominal_value=tzuicrfmiw  v_capacitor_specify=off  v_capacitor_priority=None  v_capacitor=iupzrlgfwv V  v_capacitor_nominal_specify=off  v_capacitor_nominal_unit=V  v_capacitor_nominal_value=bteppzsfbq  power_dissipated_specify=off  power_dissipated_priority=None  power_dissipated=vgtypgtqwb W  power_dissipated_nominal_specify=off  power_dissipated_nominal_unit=W  power_dissipated_nominal_value=rivyucsjkr  thermal_network_parameterization=dwdjjzljvg  Rth=nlyehmiwzy K/W  Rth_Foster=yzvtduxlms K/W  thermal_mass_parameterization=bpmvkoavun  thermal_mass=auujtwcsse J/K  thermal_mass_Foster=fcwayageqr J/K  thermal_time_constant=ugsvzufjek s  thermal_time_constant_Foster=wsnftnzmfm s  thermal_mass_initial_temperatures=volfmcadnt degC
      settings: SourceProductName=Simscape Electrical  InternalSimscapePortConfiguration="{\"Bottom\":[],\"Left\":[{\"id\":\"p\",\"label\":\"\",\"type\":\"foundation.electrical.electrical\"},{\"id\":\"H\",\"label\":\"H\",\"type\":\"foundation.thermal.thermal\"}],\"Right\":[{\"id\":\"n\",\"label\":\"\",\"type\":\"foundation.electrical.electrical\"}],\"Top\":[]}"
  Redacted_8663 : fl_lib/Electrical/Electrical Elements/Switch  R_closed=bsvpkknarh Ohm  G_open=gysxyjqdim 1/Ohm  Threshold=dsqcykyxav  i_specify=off  i_priority=None  i=niwzijarqd A  i_nominal_specify=off  i_nominal_unit=A  i_nominal_value=pvqlhifamg  v_specify=off  v_priority=None  v=rcnsccsqmx V  v_nominal_specify=off  v_nominal_unit=V  v_nominal_value=xrqqyaewad
      settings: SourceProductName=Simscape
  Redacted_4986 : PMIOPort  Side=Left
  Redacted_1147 : PMIOPort  Port=2  Side=Left
  Redacted_547 : PMIOPort  Port=3  Side=Left
  Redacted_6414 : PMIOPort  Port=4  Side=Right
  Redacted_806 : PMIOPort  Port=5  Side=Right
  Redacted_5482 : PMIOPort  Port=6  Side=Right
  Redacted_3395 : PMIOPort  Port=7  Side=Left
  Redacted_3868 : PMIOPort  Port=8  Side=Right
  connections:
  Redacted_5420/LConn1 -- Redacted_8421/LConn2 -- Redacted_5973/LConn2
  Redacted_6414/RConn1 -- Redacted_8663/RConn2
  Redacted_5973/LConn1 -- Redacted_8663/LConn1 -- Redacted_8421/RConn1
  Redacted_8421/LConn1 -- Redacted_4986/RConn1 -- Redacted_5973/RConn1
  Redacted_7227/RConn1 -- Redacted_5420/RConn1 -- Redacted_1933/RConn1 -- Redacted_7604/LConn1
  Redacted_7973/LConn1 -- Redacted_547/RConn1 -- Redacted_7937/RConn1
  Redacted_5482/RConn1 -- Redacted_7644/RConn2
  Redacted_3868/RConn1 -- Redacted_7644/RConn1 -- Redacted_6743/RConn1 -- Redacted_8663/RConn1
  Redacted_806/RConn1 -- Redacted_6743/RConn2
  Redacted_7937/LConn1 -- Redacted_7644/LConn1 -- Redacted_7973/RConn1
  Redacted_7937/LConn2 -- Redacted_1933/LConn1 -- Redacted_7973/LConn2
  Redacted_7604/RConn1 -- Redacted_3395/RConn1
  Redacted_5860/LConn2 -- Redacted_7227/LConn1
  Redacted_6743/LConn1 -- Redacted_5860/RConn1
  Redacted_5860/LConn1 -- Redacted_1147/RConn1
